simulink model "counterlogic_chida"  (R2017a)
settings: Solver=FixedStepDiscrete  StartTime=0.0  StopTime=10.0  FixedStep=0.1  RelTol=1e-3
settings Model: Creator=peram  LastModifiedBy=peram

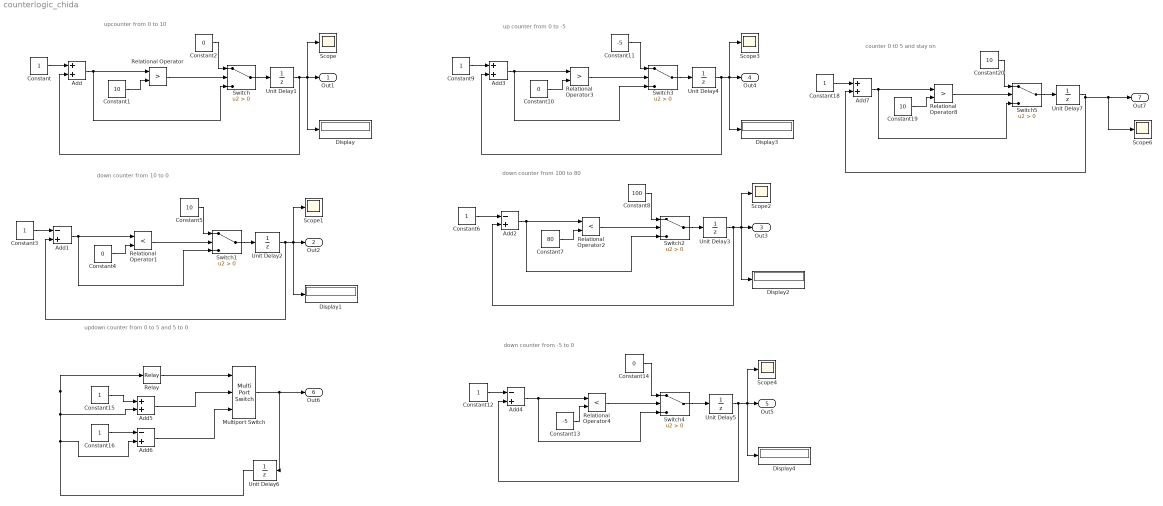
== system counterlogic_chida ==
  note: counter 0 t0 5 and stay on
  note: updown counter from 0 to 5 and 5 to 0
  note: down counter from -5 to 0
  note: up counter from 0 to -5
  note: down counter from 100 to 80
  note: upcounter from 0 to 10
  note: down counter from 10 to 0
  Add{,3,5,7} (4 alike) : Sum
  Add{1..2,4,6} (4 alike) : Sum  Inputs=-+
  Constant{,3,6,9,12,15..16,18} (8 alike) : Constant
  Constant{1,5,19..20} (4 alike) : Constant  Value=10
  Constant{2,4,10,14} (4 alike) : Constant  Value=0
  Constant11 : Constant  Value=-5
  Constant13 : Constant  Value=-5
  Constant7 : Constant  Value=80
  Constant8 : Constant  Value=100
  Display{,1..4} (5 alike) : Display
  Multiport Switch : MultiPortSwitch  DataPortOrder=Zero-based contiguous  Inputs=2
  Relational Operator : RelationalOperator  Operator=>  OutDataTypeStr=boolean  RndMeth=Simplest
  Relational Operator1 : RelationalOperator  Operator=<  OutDataTypeStr=boolean  RndMeth=Simplest
  Relational Operator2 : RelationalOperator  Operator=<  OutDataTypeStr=boolean  RndMeth=Simplest
  Relational Operator3 : RelationalOperator  Operator=>  OutDataTypeStr=boolean  RndMeth=Simplest
  Relational Operator4 : RelationalOperator  Operator=<  OutDataTypeStr=boolean  RndMeth=Simplest
  Relational Operator8 : RelationalOperator  Operator=>  OutDataTypeStr=boolean  RndMeth=Simplest
  Relay : Relay  OnSwitchValue=5  OffSwitchValue=0
  Scope{,1..4,6} (6 alike) : Scope
  Switch{,1..5} (6 alike) : Switch  Criteria=u2 > Threshold
  Unit Delay{1..7} (7 alike) : UnitDelay  SampleTime=-1
  Out1 : Outport
  Out2 : Outport  Port=2
  Out3 : Outport  Port=3
  Out4 : Outport  Port=4
  Out5 : Outport  Port=5
  Out6 : Outport  Port=6
  Out7 : Outport  Port=7
  wires:
  Constant/1 -> Add/1
  Add/1 -> Relational Operator/1, Switch/3
  Constant1/1 -> Relational Operator/2
  Relational Operator/1 -> Switch/2
  Constant2/1 -> Switch/1
  Switch/1 -> Unit Delay1/1
  Unit Delay1/1 -> Add/2, Scope/1, Display/1, Out1/1
  Switch1/1 -> Unit Delay2/1
  Relational Operator1/1 -> Switch1/2
  Constant3/1 -> Add1/1
  Unit Delay2/1 -> Add1/2, Scope1/1, Display1/1, Out2/1
  Constant4/1 -> Relational Operator1/2
  Constant5/1 -> Switch1/1
  Add1/1 -> Relational Operator1/1, Switch1/3
  Constant8/1 -> Switch2/1
  Constant7/1 -> Relational Operator2/2
  Add2/1 -> Relational Operator2/1, Switch2/3
  Switch2/1 -> Unit Delay3/1
  Constant6/1 -> Add2/1
  Relational Operator2/1 -> Switch2/2
  Unit Delay3/1 -> Add2/2, Scope2/1, Display2/1, Out3/1
  Unit Delay4/1 -> Add3/2, Scope3/1, Display3/1, Out4/1
  Constant9/1 -> Add3/1
  Relational Operator3/1 -> Switch3/2
  Switch3/1 -> Unit Delay4/1
  Constant11/1 -> Switch3/1
  Constant10/1 -> Relational Operator3/2
  Add3/1 -> Relational Operator3/1, Switch3/3
  Unit Delay5/1 -> Add4/2, Scope4/1, Display4/1, Out5/1
  Constant12/1 -> Add4/1
  Relational Operator4/1 -> Switch4/2
  Switch4/1 -> Unit Delay5/1
  Constant13/1 -> Relational Operator4/2
  Add4/1 -> Switch4/3, Relational Operator4/1
  Constant14/1 -> Switch4/1
  Relay/1 -> Multiport Switch/1
  Multiport Switch/1 -> Unit Delay6/1, Out6/1
  Constant15/1 -> Add5/1
  Add5/1 -> Multiport Switch/2
  Add6/1 -> Multiport Switch/3
  Constant16/1 -> Add6/1
  Unit Delay6/1 -> Add6/2, Add5/2, Relay/1
  Add7/1 -> Relational Operator8/1, Switch5/3
  Constant19/1 -> Relational Operator8/2
  Constant18/1 -> Add7/1
  Switch5/1 -> Unit Delay7/1
  Unit Delay7/1 -> Scope6/1, Out7/1, Add7/2
  Relational Operator8/1 -> Switch5/2
  Constant20/1 -> Switch5/1
